simulink model "PID_OpenLoop_control"  (R2025a)
settings: Solver=VariableStepAuto  StartTime=0.0  StopTime=10.0  RelTol=1e-3
InitFcn:
  | Wn = 10;
  | 
  | T = 0.001;
  | 
  | Kp = 1.5;
  | Ki = 0.2;
  | Kd = 0.001;
undefined symbols (not defined in the file): dspblkCoreblockFVToolHelper, gcbh
settings Model: Creator=星必尘Sguan  LastModifiedBy=星必尘Sguan
settings SFSimCC: SimCustomHeaderCode="#include \"PID_Loop.h\""  SimCustomInitializer=PID_Init();  SimUserSources=PID_Loop.c

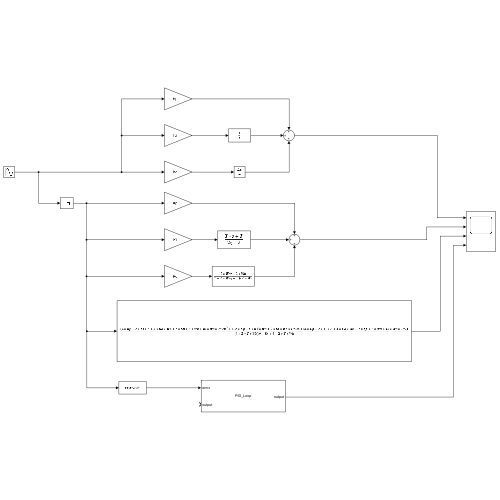
[thumbnail: Simulink's stored preview of the top-level diagram]
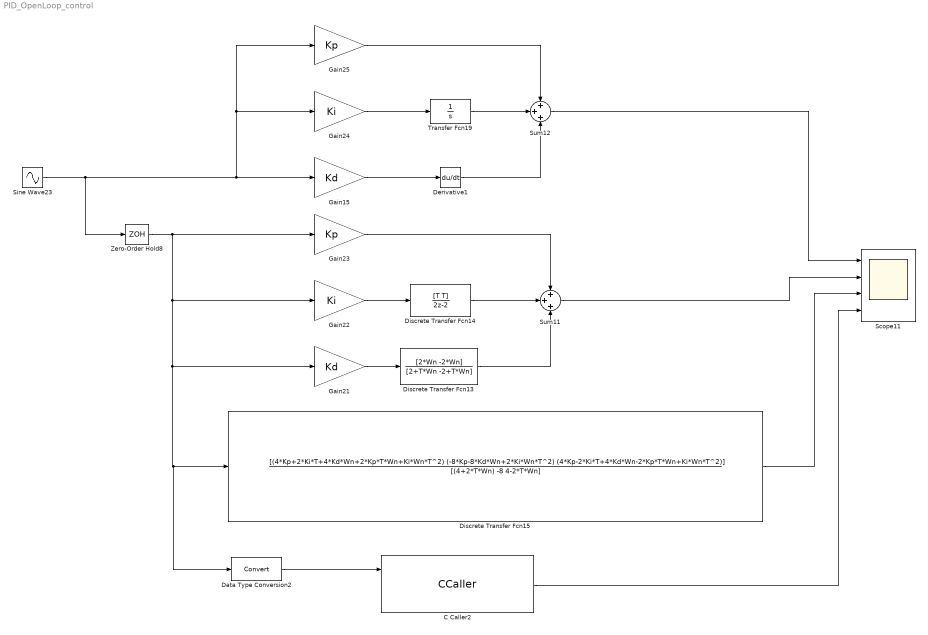
== system PID_OpenLoop_control ==
  C Caller2 : CCaller  FunctionName=PID_Loop  PortSpecificationStruct="%)30     .    X ,   8    (     @         %    \"     (    !     0         %  0 \"0    $    _    07)G3F%M90  4&]R=$YA;64 4V-O<&4     26YD97@     5'EP90      4VEZ90      27-';&]B86P   X    X    !@    @    $          4    (     0    4    !         !     %    97)R;W(    .    .     8    (    !          %    \"     $    %     0         0    !0   &5R<F]R    #@   #@    &    \"     0         !0    @    !    !0    $         $     4   !);G!U=     X    X    !@    @    &          4    (     0    $    !          D    (               .    .     8    (    !          %    \"     $    &     0         0    !@   '-I;F=L90  #@   #     &    \"     0         !0    @    !     0    $         $  ! #$    .    ,     8    (    \"0(        %    \"     $    !     0         \"  $       X    X    !@    @    $          4    (     0    8    !         !     &    ;W5T<'5T   .    .     8    (    !          %    \"     $    &     0         0    !@   &]U='!U=   #@   $     &    \"     0         !0    @    !    \"P    $         $     L   !);G!U=$]U='!U=       #@   #@    &    \"     8         !0    @    !     0    $         \"0    @           #P/PX    X    !@    @    $          4    (     0    8    !         !     &    <VEN9VQE   .    ,     8    (    !          %    \"     $    \"     0         0  ( +3$   X    P    !@    @    ) @        4    (     0    $    !          (  0"
  Data Type Conversion2 : DataTypeConversion  SaturateOnIntegerOverflow=off  RndMeth=Floor
  Derivative1 : Derivative
  Discrete Transfer Fcn13 : DiscreteTransferFcn  LoadFcn=dspblkCoreblockFVToolHelper(gcbh,'load');  Numerator=[2*Wn -2*Wn]  Denominator=[2+T*Wn -2+T*Wn]
      settings: CopyFcn=dspblkCoreblockFVToolHelper(gcbh,'copy');  DeleteFcn=dspblkCoreblockFVToolHelper(gcbh,'close');  ModelCloseFcn=dspblkCoreblockFVToolHelper(gcbh,'close');  PreSaveFcn=dspblkCoreblockFVToolHelper(gcbh,'presave');  PostSaveFcn=dspblkCoreblockFVToolHelper(gcbh,'postsave');  CloseFcn=dspblkCoreblockFVToolHelper(gcbh,'close');
  Discrete Transfer Fcn14 : DiscreteTransferFcn  LoadFcn=dspblkCoreblockFVToolHelper(gcbh,'load');  Numerator=[T T]  Denominator=[2 -2]
      settings: CopyFcn=dspblkCoreblockFVToolHelper(gcbh,'copy');  DeleteFcn=dspblkCoreblockFVToolHelper(gcbh,'close');  ModelCloseFcn=dspblkCoreblockFVToolHelper(gcbh,'close');  PreSaveFcn=dspblkCoreblockFVToolHelper(gcbh,'presave');  PostSaveFcn=dspblkCoreblockFVToolHelper(gcbh,'postsave');  CloseFcn=dspblkCoreblockFVToolHelper(gcbh,'close');
  Discrete Transfer Fcn15 : DiscreteTransferFcn  LoadFcn=dspblkCoreblockFVToolHelper(gcbh,'load');  Numerator=[(4*Kp+2*Ki*T+4*Kd*Wn+2*Kp*T*Wn+Ki*Wn*T^2) (-8*Kp-8*Kd*Wn+2*Ki*Wn*T^2) (4*Kp-2*Ki*T+4*Kd*Wn-2*Kp*T*Wn+Ki*Wn*T^2)]  Denominator=[(4+2*T*Wn) -8 4-2*T*Wn]
      settings: CopyFcn=dspblkCoreblockFVToolHelper(gcbh,'copy');  DeleteFcn=dspblkCoreblockFVToolHelper(gcbh,'close');  ModelCloseFcn=dspblkCoreblockFVToolHelper(gcbh,'close');  PreSaveFcn=dspblkCoreblockFVToolHelper(gcbh,'presave');  PostSaveFcn=dspblkCoreblockFVToolHelper(gcbh,'postsave');  CloseFcn=dspblkCoreblockFVToolHelper(gcbh,'close');
  Gain15 : Gain  Gain=Kd
  Gain21 : Gain  Gain=Kd
  Gain22 : Gain  Gain=Ki
  Gain23 : Gain  Gain=Kp
  Gain24 : Gain  Gain=Ki
  Gain25 : Gain  Gain=Kp
  Scope11 : Scope  NumInputPorts=4
      settings: ActiveDisplayYMinimum=0.057080287750086  ActiveDisplayYMaximum=3.5506703969871358  DataLoggingVariableName=ScopeData12
  Sine Wave23 : Sin  Amplitude=0.5  Bias=0.5  SampleTime=0
  Sum11 : Sum  Inputs=+++
  Sum12 : Sum  Inputs=+++
  Transfer Fcn19 : TransferFcn  Denominator=[1 0]
  Zero-Order Hold8 : ZeroOrderHold  SampleTime=0.001
  wires:
  Gain24/1 -> Transfer Fcn19/1
  Gain15/1 -> Derivative1/1
  C Caller2/1 -> Scope11/4
  Sine Wave23/1 -> Gain25/1, Gain24/1, Gain15/1, Zero-Order Hold8/1
  Zero-Order Hold8/1 -> Data Type Conversion2/1, Discrete Transfer Fcn15/1, Gain21/1, Gain22/1, Gain23/1
  Discrete Transfer Fcn15/1 -> Scope11/3
  Sum12/1 -> Scope11/1
  Gain22/1 -> Discrete Transfer Fcn14/1
  Discrete Transfer Fcn14/1 -> Sum11/2
  Sum11/1 -> Scope11/2
  Gain25/1 -> Sum12/1
  Gain23/1 -> Sum11/1
  Transfer Fcn19/1 -> Sum12/2
  Derivative1/1 -> Sum12/3
  Gain21/1 -> Discrete Transfer Fcn13/1
  Discrete Transfer Fcn13/1 -> Sum11/3
  Data Type Conversion2/1 -> C Caller2/1
